simulink model "TMR4515_DHT_FINAL"  (R2019a)
settings: Solver=ode45  StartTime=0.0  StopTime=20  FixedStep=Ts  RelTol=1e-3  EnableMultiTasking=on
values from neighbouring files (symbols this model uses):
  alfa1 = .2    (= 0.2)    [parameters.m]
  alfa2 = .2    (= 0.2)    [parameters.m]
  b1 = 0.1    [init_kalman.m]    (also in kalm.m; parameters.m)
  b2 = 0.1    [init_kalman.m]    (also in kalm.m; parameters.m)
  b3_nom = 0.1    [parameters.m]
  b4_nom = 0.1    [parameters.m]
  b5 = 0.1    [init_kalman.m]    (also in kalm.m; parameters.m)
  C = zeros(2,10)    [init_kalman.m]    (also in kalm.m)
  k1 = 0.15    [init_kalman.m]    (also in kalm.m; parameters.m)
  k3_nom = .1    (= 0.1)    [parameters.m]
  k4_nom = .1    (= 0.1)    [parameters.m]
  m1 = 1    [parameters.m]
  m2 = 1    [parameters.m]
  m3 = 1    [parameters.m]
  m4 = 1    [parameters.m]
  Qd = H22'*H12    [init_kalman.m]    (also in kalmd_COPY.m = (Qd+Qd')/2)
  Rd = R/Ts    [init_kalman.m]    (also in kalmd_COPY.m = rn/Ts)
  Ts = 0.001    [init_kalman.m]    (also in kalm.m; parameters.m)
undefined symbols (not defined in the file or in its folder): A_D_Re_GNARC, Ad, Ad_1, Ad_2, Ad_3, B_D_Re_GNARC, Bd, Bd_1, Bd_2, Bd_3, C_D_Re_GNARC, D_D_Re_GNARC, Kgain_1, Kgain_2, Kgain_3, P_1, P_2, P_3, sigbuilder_block
libraries: simulink x4
settings Model: Creator=VAHiD  LastModifiedBy=Toni
settings DataIOCC: LimitDataPoints=on  SaveFormat=Array  ReturnWorkspaceOutputs=off
settings OptimizationCC: ExpressionDepthLimit=2147483647  LifeSpan=inf
settings DebuggingCC: UnderspecifiedInitializationDetection=Classic  MergeDetectMultiDrivingBlocksExec=none  SolverPrmCheckMsg=warning  FcnCallInpInsideContextMsg=warning  StateNameClashWarn=warning  SFUnexpectedBacktrackingDiag=warning  SFNoUnconditionalDefaultTransitionDiag=warning  SFExecutionAtInitializationDiag=none  ArithmeticOperatorsInVariantConditions=warning
settings HardwareCC: ProdBitPerPointer=32  ProdBitPerSizeT=32  ProdBitPerPtrDiffT=32  ProdLargestAtomicFloat=None  ProdIntDivRoundTo=Undefined  ProdEndianess=Unspecified  ProdWordSize=32  ProdHWDeviceType=32-bit Generic
settings ModelReferenceCC: PropagateSignalLabelsOutOfModel=off
settings SFSimCC: SimUseLocalCustomCode=off
settings RTWCC: RTWUseLocalCustomCode=off
settings CodeAppCC: StateflowObjectComments=on
settings GRTTargetCC: TargetLangStandard=C89/C90 (ANSI)  GeneratePreprocessorConditionals=Disable all  CombineOutputUpdateFcns=off  GRTInterface=on
settings ConfigComp: CovMetricSettings=dw  CovHtmlReporting=on  CovSaveCumulativeToWorkspaceVar=on  CovSaveSingleToWorkspaceVar=on  CovExternalEMLEnable=off

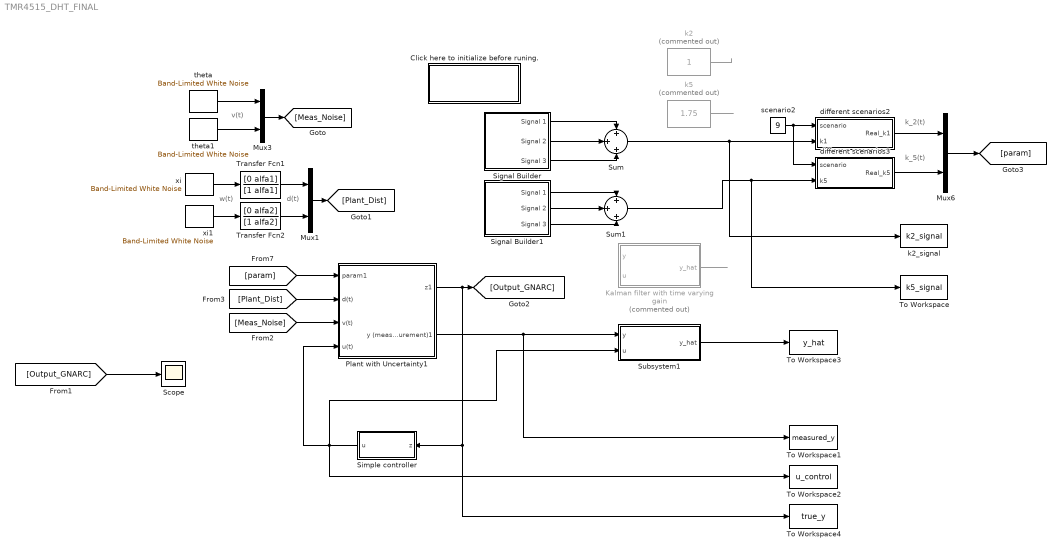
== system TMR4515_DHT_FINAL ==
  note: w(t)
  note: v(t)
  note: d(t)
  note: k_2(t)
  note: k_5(t)
  Click here to initialize before runing. : Subsystem
      settings: OpenFcn=start_up
      mask Display: disp('Load\Parameters')
  Kalman filter with time varying gain : Subsystem  Commented=on
  Mux1 : Mux  Inputs=2
  Mux3 : Mux  Inputs=2
  Mux6 : Mux  Inputs=2
  Plant with Uncertainty1 : Subsystem
  Scope : Scope
  Signal Builder : Subsystem  Tag=STV Subsys  LoadFcn=sigbuilder_block('load');  StartFcn=sigbuilder_block('start');  StopFcn=sigbuilder_block('stop');  ClipboardFcn=sigbuilder_block('clipboard');  mask(Sigbuilder block){tuvar=[0:10]}
      mask help: Simulink:masks:SigbuilderBlock_MD
      mask init:
      | if ~strcmp(get_param(bdroot(gcbh),'SimulationStatus'),'stopped') tuvar = sigbuilder_block('maskInit'); end
      settings: CopyFcn=sigbuilder_block('copy');  DeleteFcn=sigbuilder_block('delete');  ModelCloseFcn=sigbuilder_block('modelClose');  PreSaveFcn=sigbuilder_block('preSave');  PauseFcn=sigbuilder_block('pause');  ContinueFcn=sigbuilder_block('continue');  NameChangeFcn=sigbuilder_block('namechange');  OpenFcn=sigbuilder_block('open',[325.2 97.2 550.8 400.2 ]);  CloseFcn=sigbuilder_block('close');
      mask Display: plot(0, 0, 100, 100,[2, 2, 32, 32, 2], [68, 8, 8, 68, 68],[32, 2], [38, 38], [32, 19, 2],[53, 60, 44], [32, 17, 17, 2],[16, 16, 31, 31]);txt = getActiveGroup(gcbh);text(2, 100, txt,'verticalAlignment', 'top');
  Signal Builder1 : Subsystem  Tag=STV Subsys  LoadFcn=sigbuilder_block('load');  StartFcn=sigbuilder_block('start');  StopFcn=sigbuilder_block('stop');  ClipboardFcn=sigbuilder_block('clipboard');  mask(Sigbuilder block){tuvar=[0:10]}
      mask help: Simulink:masks:SigbuilderBlock_MD
      mask init:
      | if ~strcmp(get_param(bdroot(gcbh),'SimulationStatus'),'stopped') tuvar = sigbuilder_block('maskInit'); end
      settings: CopyFcn=sigbuilder_block('copy');  DeleteFcn=sigbuilder_block('delete');  ModelCloseFcn=sigbuilder_block('modelClose');  PreSaveFcn=sigbuilder_block('preSave');  PauseFcn=sigbuilder_block('pause');  ContinueFcn=sigbuilder_block('continue');  NameChangeFcn=sigbuilder_block('namechange');  OpenFcn=sigbuilder_block('open',[437.6 199.2 550.4 400 ]);  CloseFcn=sigbuilder_block('close');
      mask Display: plot(0, 0, 100, 100,[2, 2, 32, 32, 2], [68, 8, 8, 68, 68],[32, 2], [38, 38], [32, 19, 2],[53, 60, 44], [32, 17, 17, 2],[16, 16, 31, 31]);txt = getActiveGroup(gcbh);text(2, 100, txt,'verticalAlignment', 'top');
  Simple controller : Subsystem
  Subsystem1 : Subsystem
  Sum : Sum  Inputs=+|+|+
  Sum1 : Sum  Inputs=+|+|+
  To Workspace : ToWorkspace  VariableName=k5_signal  SaveFormat=Timeseries  SampleTime=-1
  To Workspace1 : ToWorkspace  VariableName=measured_y  SaveFormat=Timeseries  SampleTime=Ts
  To Workspace2 : ToWorkspace  VariableName=u_control  SaveFormat=Timeseries  SampleTime=-1
  To Workspace3 : ToWorkspace  VariableName=y_hat  SaveFormat=Timeseries  SampleTime=-1
  To Workspace4 : ToWorkspace  VariableName=true_y  SaveFormat=Timeseries  SampleTime=Ts
  Transfer Fcn1 : TransferFcn  Numerator=[0 alfa1]  Denominator=[1 alfa1]
  Transfer Fcn2 : TransferFcn  Numerator=[0 alfa2]  Denominator=[1 alfa2]
  different scenarios2 : Subsystem
  different scenarios3 : Subsystem
  k2 : Constant  Commented=on
  k2_signal : ToWorkspace  VariableName=k2_signal  SaveFormat=Timeseries  SampleTime=-1
  k5 : Constant  Commented=on  Value=1.75
  scenario2 : Constant  Value=9
  theta : simulink/Sources/Band-Limited White Noise  Cov=TH1  Ts=Ts  seed=1
  theta1 : simulink/Sources/Band-Limited White Noise  Cov=TH2  Ts=Ts  seed=2
  xi : simulink/Sources/Band-Limited White Noise  Cov=XI1  Ts=Ts  seed=3
  xi1 : simulink/Sources/Band-Limited White Noise  Cov=XI2  Ts=Ts  seed=4
  wires:
  Mux3/1 -> [Meas_Noise]
  theta/1 -> Mux3/1
  theta1/1 -> Mux3/2
  Mux1/1 -> [Plant_Dist]
  xi/1 -> Transfer Fcn1/1
  xi1/1 -> Transfer Fcn2/1
  Transfer Fcn1/1 -> Mux1/1
  Transfer Fcn2/1 -> Mux1/2
  scenario2/1 -> different scenarios2/1(scenario), different scenarios3/1(scenario)
  different scenarios3/1(Real_k5) -> Mux6/2
  different scenarios2/1(Real_k1) -> Mux6/1
  Mux6/1 -> [param]
  [param] -> Plant with Uncertainty1/1(param1)
  [Plant_Dist] -> Plant with Uncertainty1/2(d(t))
  [Meas_Noise] -> Plant with Uncertainty1/3(v(t))
  Plant with Uncertainty1/1(z1) -> To Workspace4/1, Simple controller/1(z), [Output_GNARC]
  Simple controller/1(u) -> Subsystem1/2(u), Plant with Uncertainty1/4(u(t)), To Workspace2/1
  [Output_GNARC] -> Scope/1
  Plant with Uncertainty1/2(y (measurement)1) -> Subsystem1/1(y), To Workspace1/1
  Signal Builder/2(Signal 2) -> Sum/2
  Signal Builder/1(Signal 1) -> Sum/1
  Signal Builder/3(Signal 3) -> Sum/3
  Sum/1 -> k2_signal/1, different scenarios2/2(k1)
  Signal Builder1/2(Signal 2) -> Sum1/2
  Signal Builder1/1(Signal 1) -> Sum1/1
  k2/1 -> ?
  k5/1 -> ?
  Subsystem1/1(y_hat) -> To Workspace3/1
  Signal Builder1/3(Signal 3) -> Sum1/3
  Sum1/1 -> To Workspace/1, different scenarios3/2(k5)
  Kalman filter with time varying gain/1(y_hat) -> ?

== system TMR4515_DHT_FINAL/Click here to initialize before runing. ==

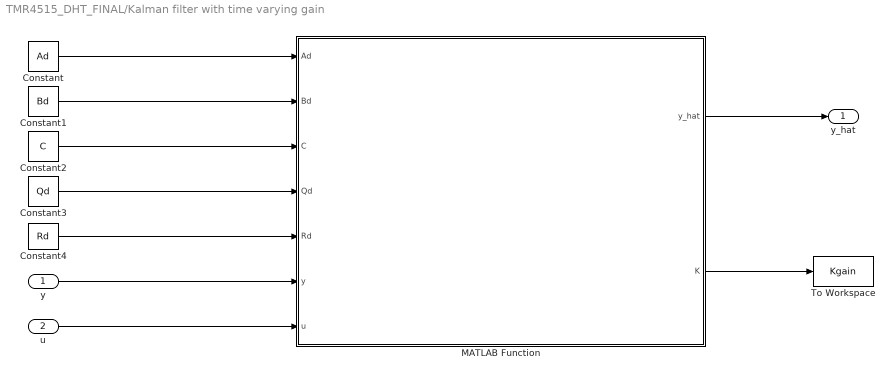
== system TMR4515_DHT_FINAL/Kalman filter with time varying gain ==
  y : Inport
  u : Inport  Port=2
  Constant : Constant  Value=Ad
  Constant1 : Constant  Value=Bd
  Constant2 : Constant  Value=C
  Constant3 : Constant  Value=Qd
  Constant4 : Constant  Value=Rd
  MATLAB Function : MATLAB Function  TreatAsAtomicUnit=on  SystemSampleTime=Ts
  To Workspace : ToWorkspace  VariableName=Kgain  SaveFormat=Timeseries  SampleTime=-1
  y_hat : Outport
  wires:
  Constant/1 -> MATLAB Function/1(Ad)
  Constant1/1 -> MATLAB Function/2(Bd)
  Constant2/1 -> MATLAB Function/3(C)
  Constant3/1 -> MATLAB Function/4(Qd)
  Constant4/1 -> MATLAB Function/5(Rd)
  MATLAB Function/1(y_hat) -> y_hat/1
  y/1 -> MATLAB Function/6(y)
  u/1 -> MATLAB Function/7(u)
  MATLAB Function/2(K) -> To Workspace/1

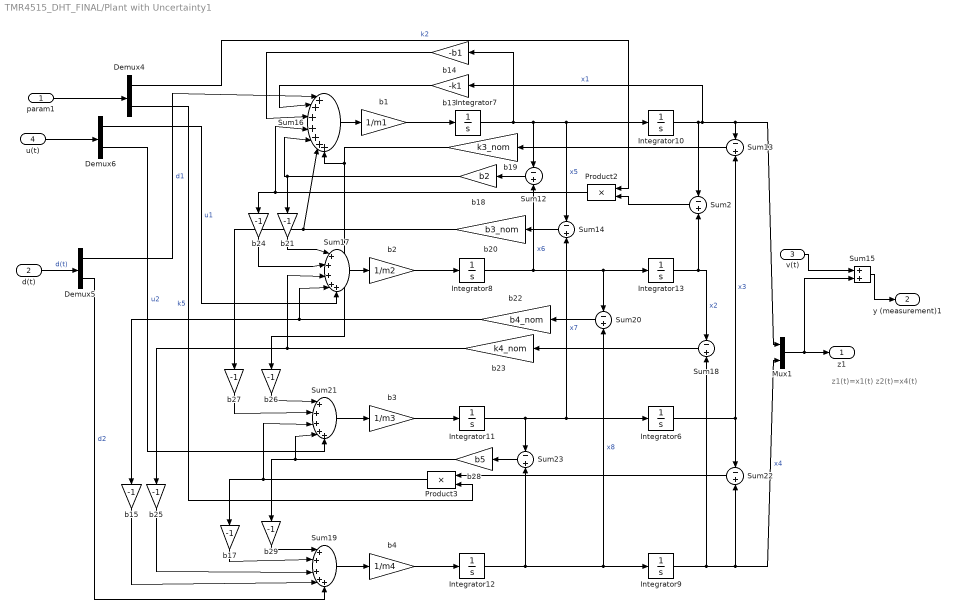
== system TMR4515_DHT_FINAL/Plant with Uncertainty1 ==
  note: z1(t)=x1(t)
      | z2(t)=x4(t)
  param1 : Inport
  d(t) : Inport  Port=2
  v(t) : Inport  Port=3
  u(t) : Inport  Port=4
  Demux4 : Demux  Outputs=2
  Demux5 : Demux  Outputs=2
  Demux6 : Demux  Outputs=2
  Integrator{6..13} (8 alike) : Integrator
  Mux1 : Mux  Inputs=2
  Product2 : Product  SaturateOnIntegerOverflow=on  InputSameDT=on  OutDataTypeStr=Inherit: Same as first input
  Product3 : Product  SaturateOnIntegerOverflow=on  InputSameDT=on  OutDataTypeStr=Inherit: Same as first input
  Sum{2,12..14,18,20,22..23} (8 alike) : Sum  Inputs=-+  SaturateOnIntegerOverflow=on  InputSameDT=on  OutDataTypeStr=Inherit: Same as first input
  Sum15 : Sum  SaturateOnIntegerOverflow=on  InputSameDT=on  OutDataTypeStr=Inherit: Same as first input
  Sum16 : Sum  Inputs=|+++++++  SaturateOnIntegerOverflow=on  InputSameDT=on  OutDataTypeStr=Inherit: Same as first input
  Sum17 : Sum  Inputs=|+++++  SaturateOnIntegerOverflow=on  InputSameDT=on  OutDataTypeStr=Inherit: Same as first input
  Sum19 : Sum  Inputs=|+++++  SaturateOnIntegerOverflow=on  InputSameDT=on  OutDataTypeStr=Inherit: Same as first input
  Sum21 : Sum  Inputs=|+++++  SaturateOnIntegerOverflow=on  InputSameDT=on  OutDataTypeStr=Inherit: Same as first input
  b1 : Gain  Gain=1/m1  SaturateOnIntegerOverflow=on  OutDataTypeStr=Inherit: Same as input  ParamDataTypeStr=Inherit: Same as input
  b13 : Gain  Gain=-k1  SaturateOnIntegerOverflow=on  OutDataTypeStr=Inherit: Same as input  ParamDataTypeStr=Inherit: Same as input
  b14 : Gain  Gain=-b1  SaturateOnIntegerOverflow=on  OutDataTypeStr=Inherit: Same as input  ParamDataTypeStr=Inherit: Same as input
  b{15,17,21,24..27,29} (8 alike) : Gain  Gain=-1  SaturateOnIntegerOverflow=on  OutDataTypeStr=Inherit: Same as input  ParamDataTypeStr=Inherit: Same as input
  b18 : Gain  Gain=b2  SaturateOnIntegerOverflow=on  OutDataTypeStr=Inherit: Same as input  ParamDataTypeStr=Inherit: Same as input
  b19 : Gain  Gain=k3_nom  SaturateOnIntegerOverflow=on  OutDataTypeStr=Inherit: Same as input  ParamDataTypeStr=Inherit: Same as input
  b2 : Gain  Gain=1/m2  SaturateOnIntegerOverflow=on  OutDataTypeStr=Inherit: Same as input  ParamDataTypeStr=Inherit: Same as input
  b20 : Gain  Gain=b3_nom  SaturateOnIntegerOverflow=on  OutDataTypeStr=Inherit: Same as input  ParamDataTypeStr=Inherit: Same as input
  b22 : Gain  Gain=b4_nom  SaturateOnIntegerOverflow=on  OutDataTypeStr=Inherit: Same as input  ParamDataTypeStr=Inherit: Same as input
  b23 : Gain  Gain=k4_nom  SaturateOnIntegerOverflow=on  OutDataTypeStr=Inherit: Same as input  ParamDataTypeStr=Inherit: Same as input
  b28 : Gain  Gain=b5  SaturateOnIntegerOverflow=on  OutDataTypeStr=Inherit: Same as input  ParamDataTypeStr=Inherit: Same as input
  b3 : Gain  Gain=1/m3  SaturateOnIntegerOverflow=on  OutDataTypeStr=Inherit: Same as input  ParamDataTypeStr=Inherit: Same as input
  b4 : Gain  Gain=1/m4  SaturateOnIntegerOverflow=on  OutDataTypeStr=Inherit: Same as input  ParamDataTypeStr=Inherit: Same as input
  z1 : Outport
  y (measurement)1 : Outport  Port=2
  wires:
  Sum15/1 -> y (measurement)1/1
  v(t)/1 -> Sum15/1
  param1/1 -> Demux4/1
  Mux1/1 -> Sum15/2, z1/1
  d(t)/1 -> Demux5/1  "d(t)"
  u(t)/1 -> Demux6/1
  b25/1 -> Sum19/3
  b15/1 -> Sum19/4
  Demux5/2 -> Sum19/5  "d2"
  Integrator7/1 -> b14/1, Sum12/1, Integrator10/1, Sum14/1  "x5"
  Integrator10/1 -> b13/1, Sum13/1, Mux1/1, Sum2/1  "x1"
  Integrator8/1 -> Sum12/2, Integrator13/1, Sum20/1  "x6"
  Integrator11/1 -> Integrator6/1, Sum14/2, Sum23/1  "x7"
  Integrator12/1 -> Integrator9/1, Sum20/2, Sum23/2  "x8"
  Demux5/1 -> Sum16/1  "d1"
  b13/1 -> Sum16/2
  b14/1 -> Sum16/3
  Integrator13/1 -> Sum2/2, Sum18/1  "x2"
  Sum2/1 -> Product2/2
  Demux4/1 -> Product2/1  "k2"
  Sum12/1 -> b18/1
  b18/1 -> Sum16/5, b21/1
  Integrator6/1 -> Sum13/2, Sum22/1  "x3"
  Sum13/1 -> b19/1
  Sum14/1 -> b20/1
  b20/1 -> Sum16/6, b27/1
  Sum16/1 -> b1/1
  Product2/1 -> Sum16/4, b24/1
  Integrator9/1 -> Sum18/2, Sum22/2, Mux1/2  "x4"
  Sum18/1 -> b23/1
  b23/1 -> Sum17/3, b25/1
  Sum17/1 -> b2/1
  Sum20/1 -> b22/1
  b22/1 -> Sum17/4, b15/1
  b21/1 -> Sum17/1
  b24/1 -> Sum17/2
  Demux6/1 -> Sum17/5  "u1"
  Sum21/1 -> b3/1
  b19/1 -> Sum16/7, b26/1
  b26/1 -> Sum21/1
  b27/1 -> Sum21/2
  Sum22/1 -> Product3/1
  Product3/1 -> Sum21/3, b17/1
  Demux4/2 -> Product3/2  "k5"
  Sum23/1 -> b28/1
  b28/1 -> Sum21/4, b29/1
  Demux6/2 -> Sum21/5  "u2"
  Sum19/1 -> b4/1
  b17/1 -> Sum19/2
  b29/1 -> Sum19/1
  b1/1 -> Integrator7/1
  b2/1 -> Integrator8/1
  b3/1 -> Integrator11/1
  b4/1 -> Integrator12/1

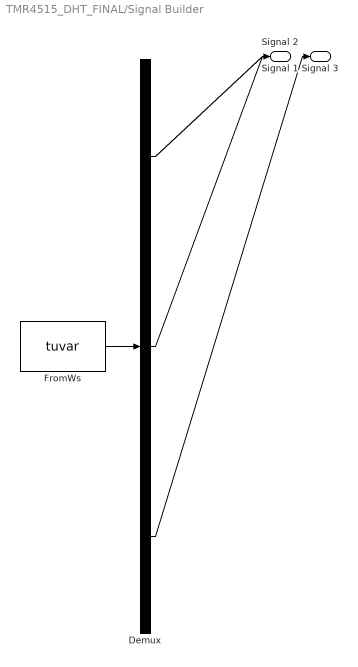
== system TMR4515_DHT_FINAL/Signal Builder ==
  Demux : Demux  Tag=STV Demux  Outputs=3
  FromWs : FromWorkspace  Tag=STV FromWs  VariableName=tuvar  SampleTime=0
      SigBuilderData=|
      | common.afterFinalStr = 'Extrapolate'
      | common.sampleTime = 0
      | dataSet.timeRange = [0 300]
      | dataSet.name = 'Group 1'
      | sbobj.Groups.Name = 'Group 1'
      | sbobj.Groups.Signals(1).Name = 'Signal 1'
      | sbobj.Groups.Signals(1).XData = [0 100 100 300]
      | sbobj.Groups.Signals(1).YData = [1 1 0 0]
      | sbobj.Groups.Signals(2).Name = 'Signal 2'
      | sbobj.Groups.Signals(2).XData = [0 100 100 200 200 300]
      | sbobj.Groups.Signals(2).YData = [0 0 2 2 0 0]
      | sbobj.Groups.Signals(3).Name = 'Signal 3'
      | sbobj.Groups.Signals(3).XData = [0 200 200 300]
      | sbobj.Groups.Signals(3).YData = [0 0 2 2]
      | sbobj.Groups.TimeRange = [0 300]
  Signal 1 : Outport  Tag=STV Outport
  Signal 2 : Outport  Tag=STV Outport  Port=2
  Signal 3 : Outport  Tag=STV Outport  Port=3
  wires:
  Demux/1 -> Signal 1/1
  Demux/2 -> Signal 2/1
  Demux/3 -> Signal 3/1
  FromWs/1 -> Demux/1

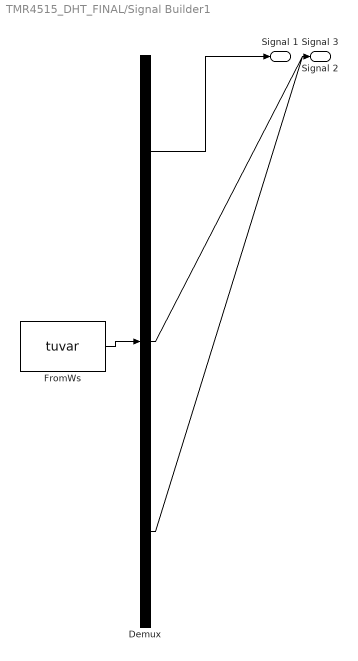
== system TMR4515_DHT_FINAL/Signal Builder1 ==
  Demux : Demux  Tag=STV Demux  Outputs=3
  FromWs : FromWorkspace  Tag=STV FromWs  VariableName=tuvar  SampleTime=0
      SigBuilderData=|
      | common.afterFinalStr = 'Extrapolate'
      | common.sampleTime = 0
      | dataSet.timeRange = [0 300]
      | dataSet.name = 'Group 1'
      | sbobj.Groups.Name = 'Group 1'
      | sbobj.Groups.Signals(1).Name = 'Signal 1'
      | sbobj.Groups.Signals(1).XData = [0 100 100 300]
      | sbobj.Groups.Signals(1).YData = [1.75 1.75 0 0]
      | sbobj.Groups.Signals(2).Name = 'Signal 2'
      | sbobj.Groups.Signals(2).XData = [0 100 100 200 200 300]
      | sbobj.Groups.Signals(2).YData = [0 0 1.25 1.25 0 0]
      | sbobj.Groups.Signals(3).Name = 'Signal 3'
      | sbobj.Groups.Signals(3).XData = [0 200 200 300]
      | sbobj.Groups.Signals(3).YData = [0 0 2 2]
      | sbobj.Groups.TimeRange = [0 300]
  Signal 1 : Outport  Tag=STV Outport
  Signal 2 : Outport  Tag=STV Outport  Port=2
  Signal 3 : Outport  Tag=STV Outport  Port=3
  wires:
  Demux/1 -> Signal 1/1
  FromWs/1 -> Demux/1
  Demux/2 -> Signal 2/1
  Demux/3 -> Signal 3/1

== system TMR4515_DHT_FINAL/Simple controller ==
  z : Inport
  Discrete mu-controller 1 : DiscreteStateSpace  Description=disp('sss')  A=A_D_Re_GNARC  B=B_D_Re_GNARC  C=C_D_Re_GNARC  D=D_D_Re_GNARC  SampleTime=Ts
  u : Outport
  wires:
  z/1 -> Discrete mu-controller 1/1
  Discrete mu-controller 1/1 -> u/1

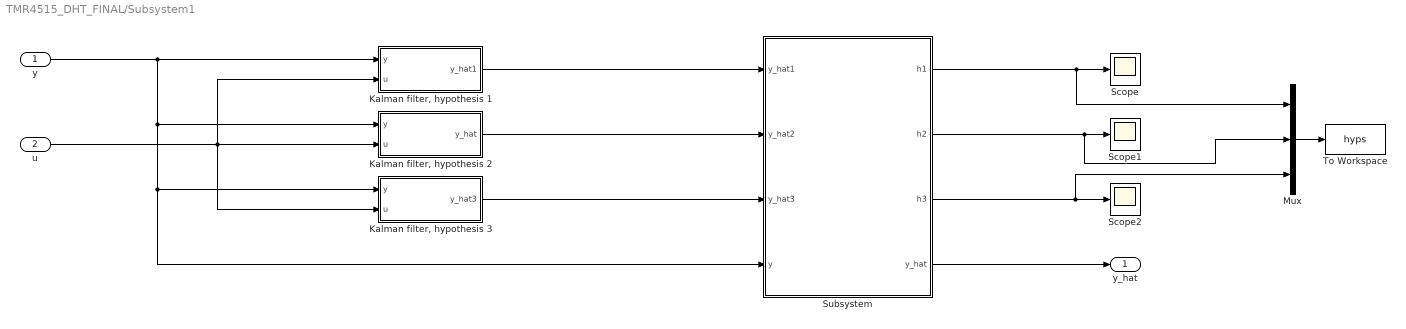
== system TMR4515_DHT_FINAL/Subsystem1 ==
  y : Inport
  u : Inport  Port=2
  "Kalman filter, hypothesis 1" : Subsystem
  "Kalman filter, hypothesis 2" : Subsystem
  "Kalman filter, hypothesis 3" : Subsystem
  Mux : Mux  Inputs=3
  Scope : Scope
  Scope1 : Scope
  Scope2 : Scope
  Subsystem : Subsystem
  To Workspace : ToWorkspace  VariableName=hyps  SaveFormat=Timeseries  SampleTime=-1
  y_hat : Outport
  wires:
  y/1 -> "Kalman filter, hypothesis 2"/1(y), Subsystem/4(y), "Kalman filter, hypothesis 3"/1(y), "Kalman filter, hypothesis 1"/1(y)
  u/1 -> "Kalman filter, hypothesis 1"/2(u), "Kalman filter, hypothesis 3"/2(u), "Kalman filter, hypothesis 2"/2(u)
  "Kalman filter, hypothesis 1"/1(y_hat1) -> Subsystem/1(y_hat1)
  "Kalman filter, hypothesis 2"/1(y_hat) -> Subsystem/2(y_hat2)
  "Kalman filter, hypothesis 3"/1(y_hat3) -> Subsystem/3(y_hat3)
  Subsystem/2(h2) -> Mux/2, Scope1/1
  Subsystem/1(h1) -> Mux/1, Scope/1
  Subsystem/3(h3) -> Mux/3, Scope2/1
  Mux/1 -> To Workspace/1
  Subsystem/4(y_hat) -> y_hat/1

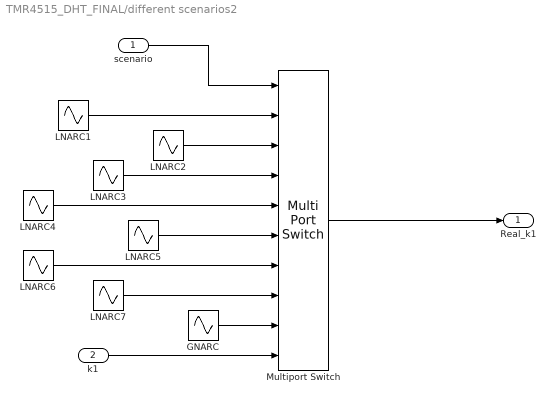
== system TMR4515_DHT_FINAL/different scenarios2 ==
  scenario : Inport
  k1 : Inport  Port=2
  GNARC : Sin  Amplitude=.75  Bias=1  Frequency=2*pi/700  Phase=-pi/2  SampleTime=0
  LNARC1 : Sin  Amplitude=.875  Bias=1.625  Frequency=2*pi/700  Phase=-pi/2  SampleTime=0
  LNARC2 : Sin  Amplitude=.55/2  Bias=.775  Frequency=2*pi/700  Phase=-pi/2  SampleTime=0
  LNARC3 : Sin  Amplitude=.75/2  Bias=1.4250  Frequency=2*pi/700  Phase=-pi/2  SampleTime=0
  LNARC4 : Sin  Amplitude=.15/2  Bias=.325  Frequency=2*pi/700  Phase=-pi/2  SampleTime=0
  LNARC5 : Sin  Amplitude=.15  Bias=.55  Frequency=2*pi/700  Phase=-pi/2  SampleTime=0
  LNARC6 : Sin  Amplitude=.45/2  Bias=.925  Frequency=2*pi/700  Phase=-pi/2  SampleTime=0
  LNARC7 : Sin  Amplitude=.30  Bias=1.45  Frequency=2*pi/700  Phase=-pi/2  SampleTime=0
  Multiport Switch : MultiPortSwitch  Inputs=9
  Real_k1 : Outport
  wires:
  Multiport Switch/1 -> Real_k1/1
  scenario/1 -> Multiport Switch/1
  LNARC3/1 -> Multiport Switch/4
  LNARC6/1 -> Multiport Switch/7
  LNARC7/1 -> Multiport Switch/8
  LNARC5/1 -> Multiport Switch/6
  LNARC4/1 -> Multiport Switch/5
  LNARC1/1 -> Multiport Switch/2
  LNARC2/1 -> Multiport Switch/3
  k1/1 -> Multiport Switch/10
  GNARC/1 -> Multiport Switch/9

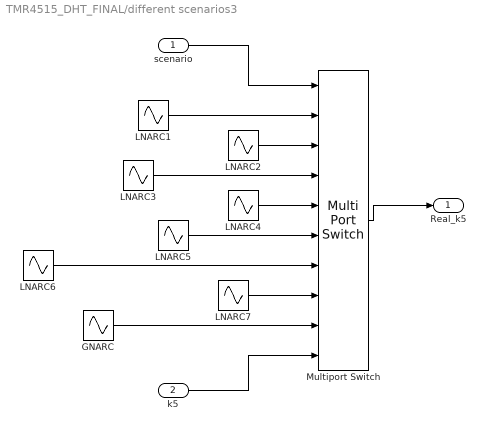
== system TMR4515_DHT_FINAL/different scenarios3 ==
  scenario : Inport
  k5 : Inport  Port=2
  GNARC : Sin  Amplitude=1.6  Bias=1.8  Frequency=2*pi/700  Phase=-pi/2  SampleTime=0
  LNARC1 : Sin  Amplitude=.8  Bias=1.7  Frequency=2*pi/700  Phase=-3*pi/2  SampleTime=0
  LNARC2 : Sin  Amplitude=.8  Bias=2.6  Frequency=2*pi/700  Phase=-pi/2  SampleTime=0
  LNARC3 : Sin  Amplitude=.8  Bias=2.6  Frequency=2*pi/700  Phase=-pi/2  SampleTime=0
  LNARC{4..7} (4 alike) : Sin  Amplitude=.8  Bias=1  Frequency=2*pi/700  Phase=-pi/2  SampleTime=0
  Multiport Switch : MultiPortSwitch  Inputs=9
  Real_k5 : Outport
  wires:
  LNARC5/1 -> Multiport Switch/6
  LNARC7/1 -> Multiport Switch/8
  LNARC6/1 -> Multiport Switch/7
  LNARC3/1 -> Multiport Switch/4
  scenario/1 -> Multiport Switch/1
  Multiport Switch/1 -> Real_k5/1
  k5/1 -> Multiport Switch/10
  GNARC/1 -> Multiport Switch/9
  LNARC1/1 -> Multiport Switch/2
  LNARC2/1 -> Multiport Switch/3
  LNARC4/1 -> Multiport Switch/5

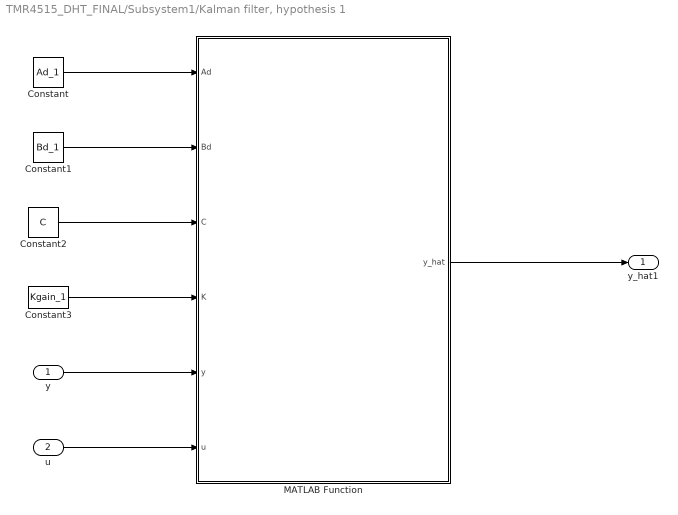
== system TMR4515_DHT_FINAL/Subsystem1/Kalman filter, hypothesis 1 ==
  y : Inport
  u : Inport  Port=2
  Constant : Constant  Value=Ad_1
  Constant1 : Constant  Value=Bd_1
  Constant2 : Constant  Value=C
  Constant3 : Constant  Value=Kgain_1
  MATLAB Function : MATLAB Function  TreatAsAtomicUnit=on  SystemSampleTime=Ts
  y_hat1 : Outport
  wires:
  Constant/1 -> MATLAB Function/1(Ad)
  Constant2/1 -> MATLAB Function/3(C)
  Constant1/1 -> MATLAB Function/2(Bd)
  MATLAB Function/1(y_hat) -> y_hat1/1
  Constant3/1 -> MATLAB Function/4(K)
  y/1 -> MATLAB Function/5(y)
  u/1 -> MATLAB Function/6(u)

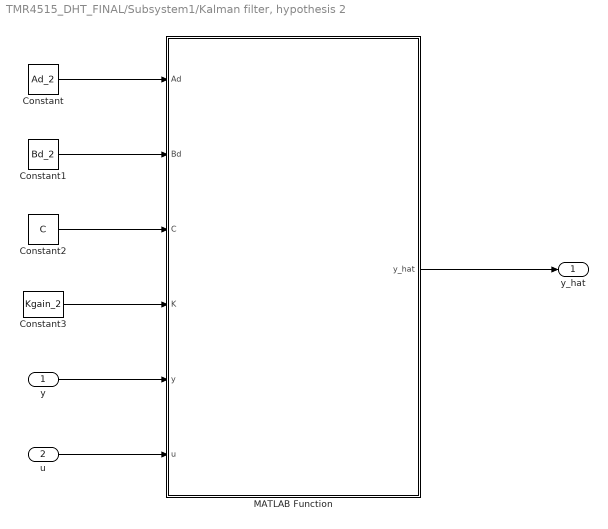
== system TMR4515_DHT_FINAL/Subsystem1/Kalman filter, hypothesis 2 ==
  y : Inport
  u : Inport  Port=2
  Constant : Constant  Value=Ad_2
  Constant1 : Constant  Value=Bd_2
  Constant2 : Constant  Value=C
  Constant3 : Constant  Value=Kgain_2
  MATLAB Function : MATLAB Function  TreatAsAtomicUnit=on  SystemSampleTime=Ts
  y_hat : Outport
  wires:
  Constant/1 -> MATLAB Function/1(Ad)
  Constant2/1 -> MATLAB Function/3(C)
  Constant1/1 -> MATLAB Function/2(Bd)
  MATLAB Function/1(y_hat) -> y_hat/1
  Constant3/1 -> MATLAB Function/4(K)
  u/1 -> MATLAB Function/6(u)
  y/1 -> MATLAB Function/5(y)

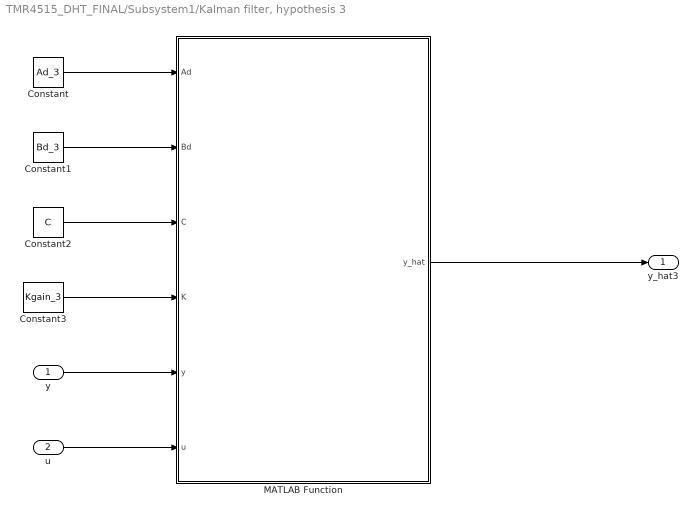
== system TMR4515_DHT_FINAL/Subsystem1/Kalman filter, hypothesis 3 ==
  y : Inport
  u : Inport  Port=2
  Constant : Constant  Value=Ad_3
  Constant1 : Constant  Value=Bd_3
  Constant2 : Constant  Value=C
  Constant3 : Constant  Value=Kgain_3
  MATLAB Function : MATLAB Function  TreatAsAtomicUnit=on  SystemSampleTime=Ts
  y_hat3 : Outport
  wires:
  Constant/1 -> MATLAB Function/1(Ad)
  Constant2/1 -> MATLAB Function/3(C)
  Constant1/1 -> MATLAB Function/2(Bd)
  MATLAB Function/1(y_hat) -> y_hat3/1
  Constant3/1 -> MATLAB Function/4(K)
  u/1 -> MATLAB Function/6(u)
  y/1 -> MATLAB Function/5(y)

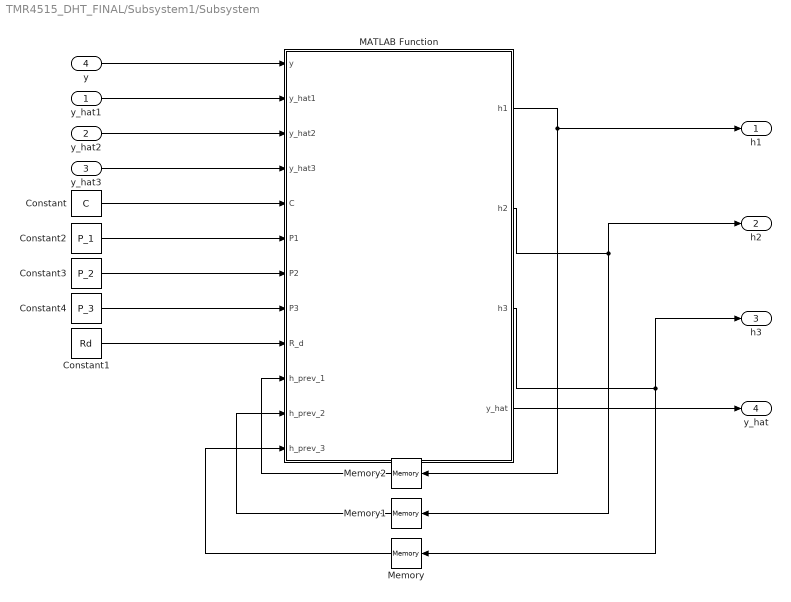
== system TMR4515_DHT_FINAL/Subsystem1/Subsystem ==
  y_hat1 : Inport
  y_hat2 : Inport  Port=2
  y_hat3 : Inport  Port=3
  y : Inport  Port=4
  Constant : Constant  Value=C
  Constant1 : Constant  Value=Rd
  Constant2 : Constant  Value=P_1
  Constant3 : Constant  Value=P_2
  Constant4 : Constant  Value=P_3
  MATLAB Function : MATLAB Function  TreatAsAtomicUnit=on  SystemSampleTime=Ts
  Memory : Memory  InitialCondition=1/3  InheritSampleTime=on
  Memory1 : Memory  InitialCondition=1/3  InheritSampleTime=on
  Memory2 : Memory  InitialCondition=1/3  InheritSampleTime=on
  h1 : Outport  VectorParamsAs1DForOutWhenUnconnected=on
  h2 : Outport  Port=2  VectorParamsAs1DForOutWhenUnconnected=on
  h3 : Outport  Port=3  VectorParamsAs1DForOutWhenUnconnected=on
  y_hat : Outport  Port=4
  wires:
  MATLAB Function/1(h1) -> Memory2/1, h1/1
  Memory2/1 -> MATLAB Function/10(h_prev_1)
  Constant1/1 -> MATLAB Function/9(R_d)
  MATLAB Function/2(h2) -> h2/1, Memory1/1
  Memory/1 -> MATLAB Function/12(h_prev_3)
  Constant/1 -> MATLAB Function/5(C)
  y_hat1/1 -> MATLAB Function/2(y_hat1)
  MATLAB Function/3(h3) -> h3/1, Memory/1
  Memory1/1 -> MATLAB Function/11(h_prev_2)
  Constant2/1 -> MATLAB Function/6(P1)
  Constant3/1 -> MATLAB Function/7(P2)
  Constant4/1 -> MATLAB Function/8(P3)
  y_hat2/1 -> MATLAB Function/3(y_hat2)
  y_hat3/1 -> MATLAB Function/4(y_hat3)
  y/1 -> MATLAB Function/1(y)
  MATLAB Function/4(y_hat) -> y_hat/1

== matlab function TMR4515_DHT_FINAL/Kalman filter with time varying gain/MATLAB Function ==
  settings: updateMethod=DISCRETE
  data: Ad input; y_hat output; Bd input; C input; Qd input; Rd input; y input; u input; K output
function [y_hat, K] = kalman(Ad,Bd,C,Qd,Rd, y, u)
% Discrete time Kalman filter 

persistent P_ x                 % error covariance and state

if isempty(P_)
    P_ = zeros(10,10);          % error covariance initialization
end

if isempty(x)
    x = zeros(10,1);            % state initialization
end

K = P_*transpose(C)*inv(C*P_*transpose(C)+Rd);                     % Kalman gain matrix


x_hat = x + K*(y-C*x);                                             % state estimate update
P_hat = (eye(10)-K*C)*P_*transpose(eye(10)-K*C)+K*Rd*transpose(K); % error covariance update

x = Ad*x_hat+Bd*u;                                                 % state estimate propagation
P_ = Ad*P_hat*transpose(Ad)+eye(10)*Qd*eye(10)';                   % error covariance propagation

y_hat = C*x;

end

== matlab function TMR4515_DHT_FINAL/Subsystem1/Kalman filter, hypothesis 2/MATLAB Function ==
  data: Ad input; Bd input; C input; K input; y input; u input; y_hat output
function y_hat = kalman(Ad,Bd,C,K, y, u)

persistent x_bar             

if isempty(x_bar)
    x_bar = zeros(10,1);           % state initialization
end

x_hat = x_bar + K*(y-C*x_bar);                                        % state estimate update
x_bar = Ad*x_hat+Bd*u;                                                % state estimate propagation

y_hat = C*x_hat;

end

== matlab function TMR4515_DHT_FINAL/Subsystem1/Kalman filter, hypothesis 1/MATLAB Function ==
  data: Ad input; Bd input; C input; K input; y input; u input; y_hat output
function y_hat = kalman(Ad,Bd,C,K, y, u)

persistent x_bar             

if isempty(x_bar)
    x_bar = zeros(10,1);           % state initialization
end

x_hat = x_bar + K*(y-C*x_bar);                                        % state estimate update
x_bar = Ad*x_hat+Bd*u;                                                % state estimate propagation

y_hat = C*x_hat;

end

== matlab function TMR4515_DHT_FINAL/Subsystem1/Kalman filter, hypothesis 3/MATLAB Function ==
  data: Ad input; Bd input; C input; K input; y input; u input; y_hat output
function y_hat = kalman(Ad,Bd,C,K, y, u)

persistent x_bar             

if isempty(x_bar)
    x_bar = zeros(10,1);           % state initialization
end

x_hat = x_bar + K*(y-C*x_bar);                                        % state estimate update
x_bar = Ad*x_hat+Bd*u;                                                % state estimate propagation

y_hat = C*x_hat;

end

== matlab function TMR4515_DHT_FINAL/Subsystem1/Subsystem/MATLAB Function ==
  data: y input; y_hat1 input; y_hat2 input; y_hat3 input; h1 output; h2 output; h3 output; C input; P1 input; P2 input; P3 input; R_d input; h_prev_1 input; h_prev_2 input; h_prev_3 input; y_hat output
function [h1, h2, h3, y_hat] = dyn_hyp(y, y_hat1,y_hat2, y_hat3, C, P1, P2, P3, R_d, h_prev_1, h_prev_2, h_prev_3)

y_tilde1 = y - y_hat1;
y_tilde2 = y - y_hat2;
y_tilde3 = y - y_hat3;
S_h1 = C*P1*C' + R_d;
S_h2 = C*P2*C' + R_d;
S_h3 = C*P3*C' + R_d;
h = zeros(1,3);
test1 = (exp(-0.5*y_tilde1'/(S_h1)*y_tilde1)/(sqrt(4*pi^2*det(S_h1))));
test2 = (exp(-0.5*y_tilde2'/(S_h2)*y_tilde2)/(sqrt(4*pi^2*det(S_h2))));
test3 = (exp(-0.5*y_tilde3'/(S_h3)*y_tilde3)/(sqrt(4*pi^2*det(S_h3))));
denominator = h_prev_1 * test1 + h_prev_2 * test2 + h_prev_3 * test3;

h(1) = (test1/denominator)*h_prev_1;
h(2) = (test2/denominator)*h_prev_2;
h(3) = (test3/denominator)*h_prev_3;

% check if any probabilities are below the threshold
for i = 1:3
    if h(i) < 5*10^(-5)
        h(i) = 5*10^(-5);
    end
end

h = h/sum(h);                       % normalize
h1 = h(1); h2 = h(2); h3 = h(3);

[~, I] = max(h);
y_hats = [y_hat1, y_hat2, y_hat3];
y_hat = y_hats(:,I);

end
